simulink subsystem "traffic_object_on_road_info"  (R2022b)
settings: Solver=VariableStepAuto  StartTime=0.0  StopTime=10.0  RelTol=1e-3
libraries: CarMaker4SL x8
settings Model: Creator=USER  LastModifiedBy=USER

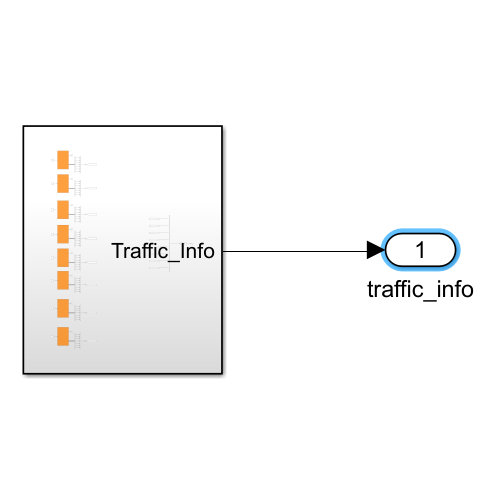
[thumbnail: Simulink's stored preview of the top-level diagram]
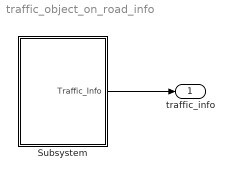
== system traffic_object_on_road_info ==
  Subsystem : Subsystem
  traffic_info : Outport
  wires:
  Subsystem/1(Traffic_Info) -> traffic_info/1

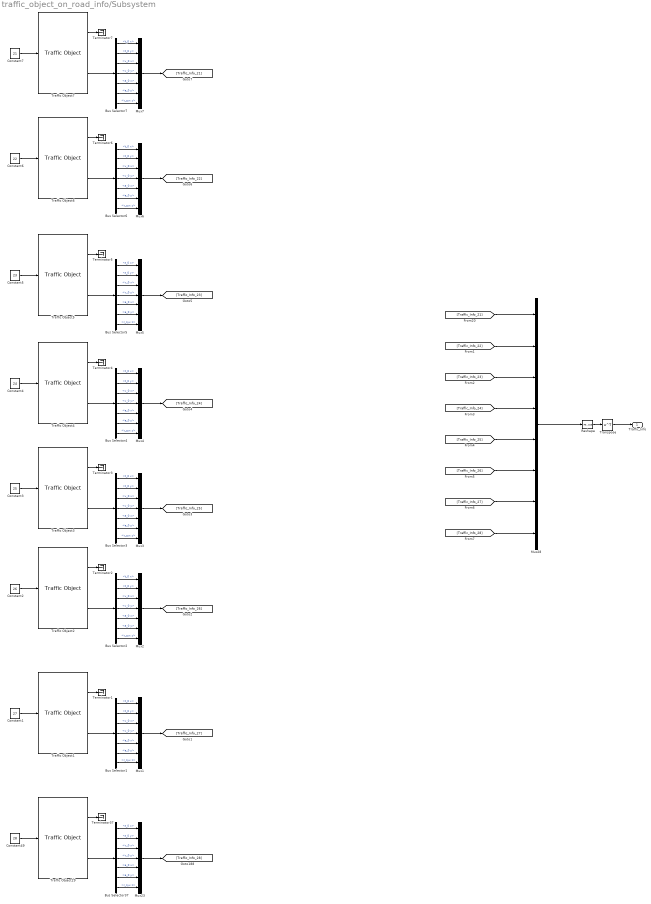
== system traffic_object_on_road_info/Subsystem ==
  Bus Selector{1..7,37} (8 alike) : BusSelector  OutputSignals=t_0 x,t_0 y,v_0 x,v_0 y,a_0 x,a_0 y,r_zyx z
  Constant1 : Constant  Value=27
  Constant2 : Constant  Value=26
  Constant3 : Constant  Value=25
  Constant4 : Constant  Value=24
  Constant49 : Constant  Value=28
  Constant5 : Constant  Value=23
  Constant6 : Constant  Value=22
  Constant7 : Constant  Value=21
  Mux{1..7,23} (8 alike) : Mux  Inputs=7
  Mux28 : Mux  Inputs=8
  Reshape : Reshape  OutputDimensionality=Customize  OutputDimensions=[7,8]
  Terminator{1..7,37} (8 alike) : Terminator
  Traffic Object1 : CarMaker4SL/Traffic Object  xname=T27  ximode=Traffic Id  xstime=Inherited
      settings: SourceProductName=CarMaker4SL
  Traffic Object2 : CarMaker4SL/Traffic Object  xname=T26  ximode=Traffic Id  xstime=Inherited
      settings: SourceProductName=CarMaker4SL
  Traffic Object29 : CarMaker4SL/Traffic Object  xname=T28  ximode=Traffic Id  xstime=Inherited
      settings: SourceProductName=CarMaker4SL
  Traffic Object3 : CarMaker4SL/Traffic Object  xname=T25  ximode=Traffic Id  xstime=Inherited
      settings: SourceProductName=CarMaker4SL
  Traffic Object4 : CarMaker4SL/Traffic Object  xname=T24  ximode=Traffic Id  xstime=Inherited
      settings: SourceProductName=CarMaker4SL
  Traffic Object5 : CarMaker4SL/Traffic Object  xname=T23  ximode=Traffic Id  xstime=Inherited
      settings: SourceProductName=CarMaker4SL
  Traffic Object6 : CarMaker4SL/Traffic Object  xname=T22  ximode=Traffic Id  xstime=Inherited
      settings: SourceProductName=CarMaker4SL
  Traffic Object7 : CarMaker4SL/Traffic Object  xname=T21  ximode=Traffic Id  xstime=Inherited
      settings: SourceProductName=CarMaker4SL
  Transpose : Math  Operator=transpose
  Traffic_Info : Outport
  wires:
  [Traffic_Info_28] -> Mux28/8
  [Traffic_Info_27] -> Mux28/7
  [Traffic_Info_26] -> Mux28/6
  [Traffic_Info_25] -> Mux28/5
  [Traffic_Info_24] -> Mux28/4
  [Traffic_Info_23] -> Mux28/3
  [Traffic_Info_22] -> Mux28/2
  Transpose/1 -> Traffic_Info/1
  Mux28/1 -> Reshape/1
  Reshape/1 -> Transpose/1
  Bus Selector7/3 -> Mux7/3  "<v_0 x>"
  Bus Selector7/1 -> Mux7/1  "<t_0 x>"
  Traffic Object7/2 -> Bus Selector7/1
  Bus Selector7/7 -> Mux7/7  "<r_zyx z>"
  Bus Selector7/6 -> Mux7/6  "<a_0 y>"
  Bus Selector7/2 -> Mux7/2  "<t_0 y>"
  Constant7/1 -> Traffic Object7/1
  Bus Selector7/5 -> Mux7/5  "<a_0 x>"
  Mux7/1 -> [Traffic_Info_21]
  Traffic Object7/1 -> Terminator7/1
  Bus Selector7/4 -> Mux7/4  "<v_0 y>"
  Bus Selector6/3 -> Mux6/3  "<v_0 x>"
  Bus Selector6/1 -> Mux6/1  "<t_0 x>"
  Traffic Object6/2 -> Bus Selector6/1
  Bus Selector6/7 -> Mux6/7  "<r_zyx z>"
  Bus Selector6/6 -> Mux6/6  "<a_0 y>"
  Bus Selector6/2 -> Mux6/2  "<t_0 y>"
  Constant6/1 -> Traffic Object6/1
  Bus Selector6/5 -> Mux6/5  "<a_0 x>"
  Mux6/1 -> [Traffic_Info_22]
  Traffic Object6/1 -> Terminator6/1
  Bus Selector6/4 -> Mux6/4  "<v_0 y>"
  Bus Selector5/3 -> Mux5/3  "<v_0 x>"
  Bus Selector5/1 -> Mux5/1  "<t_0 x>"
  Traffic Object5/2 -> Bus Selector5/1
  Bus Selector5/7 -> Mux5/7  "<r_zyx z>"
  Bus Selector5/6 -> Mux5/6  "<a_0 y>"
  Bus Selector5/2 -> Mux5/2  "<t_0 y>"
  Constant5/1 -> Traffic Object5/1
  Bus Selector5/5 -> Mux5/5  "<a_0 x>"
  Mux5/1 -> [Traffic_Info_23]
  Traffic Object5/1 -> Terminator5/1
  Bus Selector5/4 -> Mux5/4  "<v_0 y>"
  Bus Selector4/3 -> Mux4/3  "<v_0 x>"
  Bus Selector4/1 -> Mux4/1  "<t_0 x>"
  Traffic Object4/2 -> Bus Selector4/1
  Bus Selector4/7 -> Mux4/7  "<r_zyx z>"
  Bus Selector4/6 -> Mux4/6  "<a_0 y>"
  Bus Selector4/2 -> Mux4/2  "<t_0 y>"
  Constant4/1 -> Traffic Object4/1
  Bus Selector4/5 -> Mux4/5  "<a_0 x>"
  Mux4/1 -> [Traffic_Info_24]
  Traffic Object4/1 -> Terminator4/1
  Bus Selector4/4 -> Mux4/4  "<v_0 y>"
  Bus Selector3/3 -> Mux3/3  "<v_0 x>"
  Bus Selector3/1 -> Mux3/1  "<t_0 x>"
  Traffic Object3/2 -> Bus Selector3/1
  Bus Selector3/7 -> Mux3/7  "<r_zyx z>"
  Bus Selector3/6 -> Mux3/6  "<a_0 y>"
  Bus Selector3/2 -> Mux3/2  "<t_0 y>"
  Constant3/1 -> Traffic Object3/1
  Bus Selector3/5 -> Mux3/5  "<a_0 x>"
  Mux3/1 -> [Traffic_Info_25]
  Traffic Object3/1 -> Terminator3/1
  Bus Selector3/4 -> Mux3/4  "<v_0 y>"
  Bus Selector2/3 -> Mux2/3  "<v_0 x>"
  Bus Selector2/1 -> Mux2/1  "<t_0 x>"
  Traffic Object2/2 -> Bus Selector2/1
  Bus Selector2/7 -> Mux2/7  "<r_zyx z>"
  Bus Selector2/6 -> Mux2/6  "<a_0 y>"
  Bus Selector2/2 -> Mux2/2  "<t_0 y>"
  Constant2/1 -> Traffic Object2/1
  Bus Selector2/5 -> Mux2/5  "<a_0 x>"
  Mux2/1 -> [Traffic_Info_26]
  Traffic Object2/1 -> Terminator2/1
  Bus Selector2/4 -> Mux2/4  "<v_0 y>"
  Bus Selector1/3 -> Mux1/3  "<v_0 x>"
  Bus Selector1/1 -> Mux1/1  "<t_0 x>"
  Traffic Object1/2 -> Bus Selector1/1
  Bus Selector1/7 -> Mux1/7  "<r_zyx z>"
  Bus Selector1/6 -> Mux1/6  "<a_0 y>"
  Bus Selector1/2 -> Mux1/2  "<t_0 y>"
  Constant1/1 -> Traffic Object1/1
  Bus Selector1/5 -> Mux1/5  "<a_0 x>"
  Mux1/1 -> [Traffic_Info_27]
  Traffic Object1/1 -> Terminator1/1
  Bus Selector1/4 -> Mux1/4  "<v_0 y>"
  Bus Selector37/6 -> Mux23/6  "<a_0 y>"
  Bus Selector37/7 -> Mux23/7  "<r_zyx z>"
  Traffic Object29/2 -> Bus Selector37/1
  Bus Selector37/1 -> Mux23/1  "<t_0 x>"
  Bus Selector37/3 -> Mux23/3  "<v_0 x>"
  Bus Selector37/4 -> Mux23/4  "<v_0 y>"
  Traffic Object29/1 -> Terminator37/1
  Mux23/1 -> [Traffic_Info_28]
  Constant49/1 -> Traffic Object29/1
  Bus Selector37/5 -> Mux23/5  "<a_0 x>"
  Bus Selector37/2 -> Mux23/2  "<t_0 y>"
  [Traffic_Info_21] -> Mux28/1
